simulink model "ZT_VehCtrl_18B"  (R2018b)
settings: Solver=FixedStepAuto  StartTime=0.0  StopTime=inf  FixedStep=0.005  RelTol=1e-3
InitFcn:
  | mbd_mpc_consistency_checks(bdroot(gcs));
undefined symbols (not defined in the file): ANG_DEAD, BMS_NormalPwr, BrkPrsByBrkPct_TB_X, BrkPrsByBrkPct_TB_Y, DELAY_DISCHARGE, DELAY_RCUOFF, DRV_BACKWARD, DRV_BRAKE, DRV_FORWARD, DRV_NEUTRAL, DRV_PARK, DRV_UNPARK, DRV_ZEROTURN, EPB_LOCK, EPB_UNLOCK, ExtraLoadPwr, FanOff, fifo_0_vect, fifo_1_vect, HiFanReq, HV_finished, HV_No_Active, HV_POWER_OFF, HV_POWER_ON, HVDown, HVON, KaTLS_v_DrgUp_X_VehSpd, KeFTM_s_Way1OffDlyTime, KeFTM_TK_Way1CoolLv2OffBatTemp, KeFTM_TK_Way1CoolLv2OffMtrTemp, KeFTM_TK_Way1CoolLv2OnBatTemp, KeFTM_TK_Way1CoolLv2OnMtrTemp, KeFTM_TK_Way1CoolLv3OffBatTemp, KeFTM_TK_Way1CoolLv3OffMtrTemp, KeFTM_TK_Way1CoolLv3OnBatTemp, KeFTM_TK_Way1CoolLv3OnMtrTemp, KeFTM_TK_Way1CoolLv4OffBatTemp, KeFTM_TK_Way1CoolLv4OffMtrTemp, KeFTM_TK_Way1CoolLv4OnBatTemp, KeFTM_TK_Way1CoolLv4OnMtrTemp, Kp1, Kp2, LowFanReq, LQFP, MtrPwrFactor_RCU, MtrPwrHighToMidThd, MtrPwrLowToMidThd, MtrPwrMidToHighThd, MtrPwrMidToLowThd, MtrTrqMax, PCT_DEAD, Precharge, PTO_1000, PTO_540, pts1_fifo_0_vect, pts1_fifo_1_vect, pts2_fifo_0_vect, pts2_fifo_1_vect, pts3_fifo_0_vect, pts3_fifo_1_vect ... (+24)
libraries: mbd_mpc574x_ec_toolbox x124, canmsglib x72, simulink x57
(part 11 of 11)

== stateflow chart ZT_VehCtrl_18B/VehCtrl/EnergyManage1/Chart ==
  state HVon [function] [commented out]
    (default) -> (junction 44) [commented out]
    (junction 44) -> (junction 45) [commented out] : [BMS_BatteryState<=Precharge]
    (junction 44) -> (junction 46) [commented out]
    (junction 45) -> (junction 50) [commented out] : {BMS_Maincircuitcommand=HV_POWER_ON;}
    (junction 46) -> (junction 47) [commented out] : [(BMS_BatteryState==HV_finished)]
    (junction 46) -> (junction 48) [commented out] : {BMS_Maincircuitcommand=HV_No_Active;
        | BMS_Attachment1Circuit=HV_No_Active;
        | BMS_Attachment2Circuit=HV_No_Active;
        | cnt=0;}
    (junction 47) -> (junction 49) [commented out] : {BMS_Attachment1Circuit=HV_POWER_ON;
        | BMS_Attachment2Circuit=HV_POWER_ON;
        | RCU_HVOnOffSts = HVON;
        | cnt = cnt + 1;}
    (junction 49) -> (junction 48) [commented out]
    (junction 50) -> (junction 49) [commented out]
    (junction 48) -> (junction 51) [commented out]
  state PowerOff
    en,du:VCU_Maincircuitcommand = 2; cnt = cnt + 1;
    MCU_Enable = false; MCU_Discharge=true;DCDC_Enable = false;
    VCU_HVOnOffSts = HVDown;
    VCU_RexActiveDischgCmd= true;
    VCU_RexEnableCmd=false;
    VCU_RexStartStopReq=false;
    VCU_FanStsReg=0;
    VCU_MotwaterPumpDutyRe=0;
    Flag=3；
  state init
    en:Ready= false;
    VCU_Maincircuitcommand = 0;
    MCU_Enable = false; MCU_Discharge=false; DCDC_Enable = false;
    VCU_HVOnOffSts = HVON;
    VCU_RexActiveDischgCmd= false;
    VCU_RexEnableCmd=false;
    VCU_RexStartStopReq=false;
    VCU_FanStsReg=0;
    VCU_MotwaterPumpDutyRe=0;
    Flag=0;
  state PowerOn
    state BatChrgSt
      state Discharge
        en,du:
        Flag=5;cnt=cnt+1;
        Ready=false;
        DCDC_Enable = true;
        VCU_RexStartStopReq = false;
        VCU_ReqRexGenPwr = 0;
        VCU_RexEnableCmd= false;
        MCU_Enable = false;
        MCU_Discharge=true;
      state BatChrg
        en,du:
        Flag=6;
        Ready=false;
        DCDC_Enable = true;
        VCU_RexStartStopReq = false;
        VCU_ReqRexGenPwr = 0;
        VCU_RexEnableCmd= false;
        MCU_Enable = false;
        MCU_Discharge=false;
      (default) -> Discharge
      Discharge -> BatChrg : [cnt>DELAY_DISCHARGE]
    state HV_ON
      en:VCU_Maincircuitcommand = 1;
      Flag=1；
    state READY
      en:Ready=true;MCU_Enable = true; DCDC_Enable = true; Flag=2；
      VCU_RexStartStopReq = false;
      VCU_ReqRexGenPwr = 0;
      VCU_RexEnableCmd= false;
    state RCU
      state RCUAuto
        en:Flag=4;VCU_RexStartStopReq = false;
        VCU_ReqRexGenPwr = 0;
        VCU_RexEnableCmd= true;%默认不启动
        du:RcuAuto();
      state RCUOn
        en:Flag=3;
        du:VCU_RexEnableCmd= true;
        VCU_RexStartStopReq=true;
        VCU_ReqRexGenPwr = RCU_RexGenPwr;
        RcuCool();
      (default) -> RCUAuto
      RCUOn -> RCUAuto : [Rcuswitch==0]
      RCUAuto -> RCUOn : [Rcuswitch==1]
    (default) -> HV_ON
    HV_ON -> READY : [BMS_BatteryState==3]
    READY -> BatChrgSt [order 1] : [ChrgSig==1]{cnt = 0;}
    BatChrgSt -> READY : [ChrgSig==0]
    READY -> RCU [order 2] : [(RCU_RexSelfChkSt > 0) && (RCU_RexFltLvl==0)&&(Rcuswitch==0||Rcuswitch==1)]
    RCU -> READY [order 1] : [Rcuswitch==2]
    RCU -> BatChrgSt [order 2] : [ChrgSig==1]{cnt = 0;}
  state HVdown [function] [commented out]
    (default) -> (junction 157) [commented out]
    (junction 157) -> (junction 156) [commented out] : [cnt<DELAY_RCUOFF]
    (junction 157) -> (junction 155) [commented out]
    (junction 156) -> (junction 154) [commented out] : {RCU_RexEnableCmd = false;
        | MCU_Enable = false;
        | DCDC_Enable = false;
        | DCAC_Enable = false;}
    (junction 155) -> (junction 170) [commented out] : [cnt<DELAY_RCUOFF*2]
    (junction 155) -> (junction 168) [commented out] : {MCU_Discharge = true;
        | RCU_RexActiveDischgCmd = true;}
    (junction 170) -> (junction 171) [commented out] : {BMS_Maincircuitcommand=HV_POWER_OFF;
        | BMS_Attachment1Circuit=HV_POWER_OFF;
        | BMS_Attachment2Circuit=HV_POWER_OFF;}
    (junction 171) -> (junction 168) [commented out]
    (junction 154) -> (junction 171) [commented out]
    (junction 168) -> (junction 176) [commented out]
  state RcuAuto [function]
    (default) -> (junction 75) : {VCU_RexEnableCmd= true;} % 高压使能
    (junction 75) -> (junction 76) [order 1] : [(BMS_SOC<35) || (MCU_TotalPwrCmd > BMS_NormalPwr)] % 超功率或亏电，则启动增程器
    (junction 75) -> (junction 78) [order 2]
    (junction 76) -> (junction 74) : {VCU_RexStartStopReq = true;
        |  VCU_ReqRexGenPwr = RCU_RexGenPwr;}
    (junction 78) -> (junction 79) [order 1] : [(BMS_SOC>60) && (MCU_TotalPwrCmd < BMS_NormalPwr)] % 电量充足或低功率，则关闭增程器
    (junction 78) -> (junction 70) [order 2]
    (junction 79) -> (junction 80) : {VCU_RexStartStopReq = false;
        | VCU_ReqRexGenPwr = 0;}
    (junction 80) -> (junction 70)
    (junction 74) -> (junction 80)
    (junction 70) -> (junction 116) : {VCU_MotwaterPumpDutyRe = 100;} % 水泵默认工作
    (junction 116) -> (junction 118) [order 1] : [(RCU_GCUISGInverterTempHiAlarm>0) && (RCU_GCUISGMotorTempHiAlarm>0)] % 双过温，则高速风扇
    (junction 116) -> (junction 128) [order 2]
    (junction 118) -> (junction 126) : {VCU_FanStsReg = HiFanReq;}
    (junction 128) -> (junction 122) [order 1] : [(RCU_GCUISGInverterTempHiAlarm>0) || (RCU_GCUISGMotorTempHiAlarm>0)] % 单过温，则低速风扇
    (junction 128) -> (junction 121) [order 2] : {VCU_FanStsReg = FanOff;} % 未过温，则关闭风扇
    (junction 122) -> (junction 125) : {VCU_FanStsReg = LowFanReq;}
    (junction 125) -> (junction 121)
    (junction 126) -> (junction 125)
    (junction 121) -> (junction 130)
  state RcuCool [function]
    (default) -> (junction 269) : {VCU_MotwaterPumpDutyRe = 100;} % 水泵默认工作
    (junction 269) -> (junction 270) [order 1] : [(RCU_GCUISGInverterTempHiAlarm>0) && (RCU_GCUISGMotorTempHiAlarm>0)] % 双过温，则高速风扇
    (junction 269) -> (junction 271) [order 2]
    (junction 270) -> (junction 275) : {VCU_FanStsReg = HiFanReq;}
    (junction 271) -> (junction 272) [order 1] : [(RCU_GCUISGInverterTempHiAlarm>0) || (RCU_GCUISGMotorTempHiAlarm>0)] % 单过温，则低速风扇
    (junction 271) -> (junction 273) [order 2] : {VCU_FanStsReg = FanOff;} % 未过温，则关闭风扇
    (junction 272) -> (junction 274) : {VCU_FanStsReg = LowFanReq;}
    (junction 274) -> (junction 273)
    (junction 275) -> (junction 274)
    (junction 273) -> (junction 276)
  (default) -> init
  PowerOff -> init : [(cnt>DELAY_DISCHARGE)&&(BMS_BatteryState==4)]
  init -> PowerOn : [(Key>0) && ShutDown==0]
  PowerOn -> PowerOff : [(Key==0) || ShutDown>0]{cnt = 0;}
  data: Key input; ShutDown input; HV_No_Active parameter double; HV_POWER_ON parameter; HV_POWER_OFF parameter; cnt local single =single(0); VCU_Maincircuitcommand output uint8; VCU_HVOnOffSts output uint8; VCU_RexEnableCmd output boolean; VCU_RexStartStopReq output boolean; VCU_ReqRexGenPwr output single =single(-60); VCU_FanStsReg output uint8; VCU_MotwaterPumpDutyRe output single; VCU_RexActiveDischgCmd output boolean; HVON parameter; HVDown parameter; FanOff parameter; LowFanReq parameter; RCU_RexSelfChkSt input; RCU_RexFltLvl input; RCU_RexGenPwrMaxLim input; RCU_GCUISGInverterTempHiAlarm input; RCU_GCUISGMotorTempHiAlarm input; MCU_TotalPwrCmd input; HiFanReq parameter; DELAY_RCUOFF parameter; DELAY_DISCHARGE parameter; MCU_Enable output boolean; MCU_Discharge output boolean; BMS_SOC input; BMS_NormalPwr parameter; BMS_BatteryState input; ChrgSig input; Ready output; DCDC_Enable output; Precharge parameter; HV_finished parameter; Flag output; Rcuswitch input; MtrPwrHighToMidThd parameter; MtrPwrLowToMidThd parameter; MtrPwrMidToHighThd parameter; MtrPwrMidToLowThd parameter; RexGenPwrHigh parameter; RexGenPwrLow parameter; RexGenPwrMid parameter; RCU_RexGenPwr input

== stateflow chart ZT_VehCtrl_18B/VehCtrl/FaultProc/Subsystem5/TimeOutLevel_RMT1 ==
  state on
    en:TimeOutLevel=1;LifeTemp=LiveCounter;
    du:LifeTemp=LiveCounter;
  state on_cnt
    en:TimeOutLevel=1;cnt=0;
    du:cnt = cnt + 1;
  state off
    en:TimeOutLevel=0;
  (default) -> on
  on -> on_cnt : [LiveCounter==LifeTemp]
  on_cnt -> on [order 2] : [LiveCounter~=LifeTemp]
  off -> on : [LiveCounter~=LifeTemp]
  on_cnt -> off [order 1] : [(cnt>=10)]
  data: LiveCounter input; TimeOutLevel output; LifeTemp local; cnt local

== stateflow chart ZT_VehCtrl_18B/VehCtrl/FaultProc/Subsystem5/PacketLoss_RMT ==
  state on
    en:PacketLossFlg=0;
  state on_cnt
    en:PacketLossFlg=0;cnt=0;
    du:cnt = cnt + 1;
  state off
    en:PacketLossFlg=1;
  (default) -> on
  on -> on_cnt : [(PacketLoss==1)||(CheckSum==1)]
  on_cnt -> on [order 2] : [(PacketLoss==0)&(CheckSum==0)]
  off -> on : [(PacketLoss==0)&(CheckSum==0)]
  on_cnt -> off [order 1] : [(cnt>=10)]
  data: CheckSum input; PacketLossFlg output; cnt local; PacketLoss input

== stateflow chart ZT_VehCtrl_18B/VehCtrl/FaultProc/Subsystem5/PacketLoss_RMT1 ==
  state on
    en:PacketLossFlg=0;
  state on_cnt
    en:PacketLossFlg=0;cnt=0;
    du:cnt = cnt + 1;
  state off
    en:PacketLossFlg=1;
  (default) -> on
  on -> on_cnt : [(PacketLoss==1)||(CheckSum==1)]
  on_cnt -> on [order 2] : [(PacketLoss==0)&(CheckSum==0)]
  off -> on : [(PacketLoss==0)&(CheckSum==0)]
  on_cnt -> off [order 1] : [(cnt>=10)]
  data: CheckSum input; PacketLossFlg output; cnt local; PacketLoss input

== stateflow chart ZT_VehCtrl_18B/VehCtrl/FaultProc/Subsystem5/TimeOutLevel_RMT ==
  state on
    en:TimeOutLevel=1;LifeTemp=LiveCounter;
    du:LifeTemp=LiveCounter;
  state on_cnt
    en:TimeOutLevel=1;cnt=0;
    du:cnt = cnt + 1;
  state off
    en:TimeOutLevel=0;
  (default) -> on
  on -> on_cnt : [LiveCounter==LifeTemp]
  on_cnt -> on [order 2] : [LiveCounter~=LifeTemp]
  off -> on : [LiveCounter~=LifeTemp]
  on_cnt -> off [order 1] : [(cnt>=10)]
  data: LiveCounter input; TimeOutLevel output; LifeTemp local; cnt local

== stateflow chart ZT_VehCtrl_18B/SigOut/GPIO /PWM_OUT/FreqCMD ==
  settings: executeAtInitialization=1
  state A
    du:
    freq = 20000;
    cntr = cntr + 1;
    dc = 0.25;
  state A1
    du:
    freq = 10000;
    cntr = cntr - 1;
    dc =  0.5;
  (default) -> A : {cntr=0;dc=0;}
  A1 -> A : [cntr < 1]
  A -> A1 : [cntr > 50]
  data: cntr local uint32 =0; freq output uint32; dc output single

== stateflow chart ZT_VehCtrl_18B/VehCtrl/TempertureControl/ThermFR_RRvRead1/Way1_Cool_Level ==
  settings: executeAtInitialization=1
  state Ready
    state Level_1
      en:
      MtrPumpLv=1;
      Fan_Low=0;
    state Level_2
      en:
      MtrPumpLv=2;
      Fan_Low=1;
    state Level_4
      en:
      MtrPumpLv=4;
      Fan_Low=0;
    state Level_3
      en:
      MtrPumpLv=3;
      Fan_Low=1;
    Level_1 -> Level_2 : [Temp>=Ke_Lv2OnTemp]
    (default) -> Level_1
    Level_2 -> Level_1 [order 1] : [Temp<=Ke_Lv2OffTemp]
    Level_2 -> Level_3 [order 2] : [Temp>=Ke_Lv3OnTemp]
    Level_3 -> Level_2 [order 1] : [Temp<=Ke_Lv3OffTemp]
    Level_3 -> Level_4 [order 2] : [Temp>=Ke_Lv4OnTemp]
    Level_4 -> Level_3 : [Temp<=Ke_Lv4OffTemp]
  state Level_0
    en:
    MtrPumpLv=0;
    Fan_Low=0;
  state OFF_Cnt
    en:
    Cnt=1;
    du:
    Cnt++;
  (default) -> Level_0
  Level_0 -> Ready : [RdySt==1]
  OFF_Cnt -> Level_0 : [Cnt>=Ke_OffDlyCnt]
  Ready -> OFF_Cnt : [RdySt==0]
  data: RdySt input; Temp input; Ke_Lv2OffTemp input; Ke_Lv2OnTemp input; Ke_Lv3OffTemp input; Ke_Lv3OnTemp input; Ke_Lv4OffTemp input; Ke_Lv4OnTemp input; Ke_OffDlyCnt input; Cnt local uint32; Fan_Low output uint8; MtrPumpLv output double

== stateflow chart ZT_VehCtrl_18B/Initialization & SPI timer1/CS1 LS/Chart ==
  state clear
    en:high=128+7;low=1;cnt=0;
    du:cnt = cnt + 1;
  state en
    en:high=128+1+64;low=0;cnt=0;
    du:cnt = cnt + 1;
  state config
    en:high=128+7+64;low=1+128;cnt=0;
    du:cnt = cnt + 1;
  (default) -> clear
  clear -> en : [cnt>5]
  en -> config : [cnt>5]
  data: high output; low output; cnt local

== stateflow chart ZT_VehCtrl_18B/VehCtrl/TempertureControl/ThermLvRead3/Way1_Cool_Level ==
  settings: executeAtInitialization=1
  state Ready
    state Level_2
      en:
      MtrPumpLv=2;
      Fan_Low=1;
      Fan_High=0;
      V1 = 1; V2 = 1; V3 = 0; V4 = 0;
    state Level_1
      en:
      MtrPumpLv=1;
      Fan_Low=0;
      Fan_High=0;
      V1 = 1; V2 = 0; V3 = 0; V4 = 0;
    state Level_4
      en:
      MtrPumpLv=4;
      Fan_Low=0;
      Fan_High=1;
      V1 = 1; V2 = 1; V3 = 1; V4 = 1;
    state Level_3
      en:
      MtrPumpLv=3;
      Fan_Low=0;
      Fan_High=1;
      V1 = 1; V2 = 1; V3 = 1; V4 = 0;
    Level_1 -> Level_2 : [Temp>=Ke_Lv2OnTemp]
    (default) -> Level_1
    Level_2 -> Level_1 [order 1] : [Temp<=Ke_Lv2OffTemp]
    Level_2 -> Level_3 [order 2] : [Temp>=Ke_Lv3OnTemp]
    Level_3 -> Level_2 [order 1] : [Temp<=Ke_Lv3OffTemp]
    Level_3 -> Level_4 [order 2] : [Temp>=Ke_Lv4OnTemp]
    Level_4 -> Level_3 : [Temp<=Ke_Lv4OffTemp]
  state Level_0
    en:
    MtrPumpLv=0;
    Fan_Low=0;
    Fan_High=0;
    V1 = 0; V2 = 0; V3 = 0; V4 = 0;
  state OFF_Cnt
    en:
    Cnt=1;
    du:
    Cnt++;
  (default) -> Level_0
  Level_0 -> Ready : [RdySt==1]
  OFF_Cnt -> Level_0 : [Cnt>=Ke_OffDlyCnt]
  Ready -> OFF_Cnt : [RdySt==0]
  data: RdySt input; Temp input; Ke_Lv2OffTemp input; Ke_Lv2OnTemp input; Ke_Lv3OffTemp input; Ke_Lv3OnTemp input; Ke_Lv4OffTemp input; Ke_Lv4OnTemp input; Ke_OffDlyCnt input; Cnt local uint32; Fan_Low output uint8; Fan_High output uint8; V1 output double; V2 output double; V3 output double; V4 output double; MtrPumpLv output uint8

== stateflow chart ZT_VehCtrl_18B/VehCtrl/LedControl/Chart ==
  state Normal
    state Turn_Right
      state LightOn
        Right_Cmd=1;
      state LightOff
        Right_Cmd=0;
      (default) -> Normal.Turn_Right.LightOn
      Normal.Turn_Right.LightOff -> Normal.Turn_Right.LightOn : [after(0.5,sec)]
      Normal.Turn_Right.LightOn -> Normal.Turn_Right.LightOff : [after(0.5,sec)]
    state Neutral
      en:
      Left_Cmd=0;
      Right_Cmd=0;
    state Turn_Left
      state LightOn
        Left_Cmd=1;
      state LightOff
        Left_Cmd=0;
      (default) -> Normal.Turn_Left.LightOn
      Normal.Turn_Left.LightOff -> Normal.Turn_Left.LightOn : [after(0.5,sec)]
      Normal.Turn_Left.LightOn -> Normal.Turn_Left.LightOff : [after(0.5,sec)]
    Neutral -> Turn_Right [order 1] : [SteerAng>=DeadBand1]
    (default) -> Neutral
    Turn_Right -> Neutral : [SteerAng<DeadBand2]
    Turn_Left -> Neutral : [SteerAng>-DeadBand2]
    Neutral -> Turn_Left [order 2] : [SteerAng<=-DeadBand1]
  state SOCmode
    state LightOn
      Right_Cmd=1;
      Left_Cmd=1;
    state LightOff
      Right_Cmd=0;
      Left_Cmd=0;
    (default) -> SOCmode.LightOn
    SOCmode.LightOff -> SOCmode.LightOn : [after(0.5,sec)]
    SOCmode.LightOn -> SOCmode.LightOff : [after(0.5,sec)]
  (default) -> Normal
  SOCmode -> Normal : [soc>35]
  Normal -> SOCmode : [soc<30]
  data: soc input; SteerAng input; DeadBand1 local =3; DeadBand2 local =2; Left_Cmd output; Right_Cmd output

== stateflow chart ZT_VehCtrl_18B/Initialization & SPI timer1/CS3 LS/Chart ==
  state ConfigA
    en:high=80+mode*(1+4);low=0+mode*(1+4);cnt=0;
    du:cnt = cnt + 1;
  state en
    en:high=96;low=0;cnt=0;
  (default) -> ConfigA
  ConfigA -> en : [cnt>4]
  data: high output; low output; cnt local; mode input

== stateflow chart ZT_VehCtrl_18B/VehCtrl/TempertureControl/ThermFR_RRvRead2/Way1_Cool_Level ==
  settings: executeAtInitialization=1
  state Ready
    state Level_1
      en:
      MtrPumpLv=1;
      Fan_Low=0;
    state Level_2
      en:
      MtrPumpLv=2;
      Fan_Low=1;
    state Level_4
      en:
      MtrPumpLv=4;
      Fan_Low=0;
    state Level_3
      en:
      MtrPumpLv=3;
      Fan_Low=1;
    Level_1 -> Level_2 : [Temp>=Ke_Lv2OnTemp]
    (default) -> Level_1
    Level_2 -> Level_1 [order 1] : [Temp<=Ke_Lv2OffTemp]
    Level_2 -> Level_3 [order 2] : [Temp>=Ke_Lv3OnTemp]
    Level_3 -> Level_2 [order 1] : [Temp<=Ke_Lv3OffTemp]
    Level_3 -> Level_4 [order 2] : [Temp>=Ke_Lv4OnTemp]
    Level_4 -> Level_3 : [Temp<=Ke_Lv4OffTemp]
  state Level_0
    en:
    MtrPumpLv=0;
    Fan_Low=0;
  state OFF_Cnt
    en:
    Cnt=1;
    du:
    Cnt++;
  (default) -> Level_0
  Level_0 -> Ready : [RdySt==1]
  OFF_Cnt -> Level_0 : [Cnt>=Ke_OffDlyCnt]
  Ready -> OFF_Cnt : [RdySt==0]
  data: RdySt input; Temp input; Ke_Lv2OffTemp input; Ke_Lv2OnTemp input; Ke_Lv3OffTemp input; Ke_Lv3OnTemp input; Ke_Lv4OffTemp input; Ke_Lv4OnTemp input; Ke_OffDlyCnt input; Cnt local uint32; Fan_Low output uint8; MtrPumpLv output double

== stateflow chart ZT_VehCtrl_18B/VehCtrl/LedControl/Chart1 ==
  state unNormal
    en,du:Green=0;Red=1；
  state Normal
    state RMT
      en,du:Green=1;Red=0;
    state Auto
      en,du:Green=1;Red=1;%黄色
    (default) -> RMT
    RMT -> Auto : [CtrMode==1]
    Auto -> RMT : [CtrMode==0]
  (default) -> Normal
  Normal -> unNormal : [Fault>0]
  unNormal -> Normal : [Fault==0]
  data: CtrMode input; Fault input; Red output; Green output

== stateflow chart ZT_VehCtrl_18B/VehCtrl/MontionControl/ValveControl/SteerSys/Chart ==
  state Left
    en,du:flg=1;
  state Hold
    en,du:flg=0;
  state Right
    en,du:flg=2;
  (default) -> Hold
  Hold -> Left [order 1] : [StrErr>0.7]
  Left -> Hold : [StrErr<=0.5]
  Hold -> Right [order 2] : [StrErr<-0.7]
  Right -> Hold : [StrErr>-0.4]
  data: StrErr input; flg output

== stateflow chart ZT_VehCtrl_18B/VehCtrl/MontionControl/DriveControl/DriveModeTrans ==
  state Park [commented out]
    en,du:VehDrv=0;SpdTgt=0;VehBrk=CmdBrk;
    state Lock [commented out]
      en,du:EpbSt = EPB_LOCK;DrvPhase = DRV_PARK;cnt=0;
    state Unlock [commented out]
      en:EpbSt = EPB_UNLOCK;DrvPhase = DRV_UNPARK;cnt=0;
      du:VehBrk=CmdBrk;cnt = cnt + 1;
    (default) -> Lock [commented out]
    Lock -> Unlock [commented out] : [(CmdPark==EPB_UNLOCK)...
        |  || ((CmdDrv>PCT_DEAD)&&(CmdBrk<=0.5*PCT_DEAD))...
        |  || (CmdSpd>SPD_DEAD)]
        | % 释放驻车请求，或踩油门，或车速请求
    Unlock -> Lock [commented out] : [(CmdPark==EPB_LOCK)]
        | % 驻车请求
  state Run
    state TrqCtrl
      en:VehBrk=0;ModeSpd=false;SpdTgt=0;
      state Normal
        state Backward
          en,du:VehDrv=CmdDrv;DrvPhase = DRV_BACKWARD;
        state Forward
          en,du:VehDrv=CmdDrv;DrvPhase = DRV_FORWARD;
        state Neutral
          en:VehDrv=0;DrvPhase = DRV_NEUTRAL; % 预留再生制动
        Run.TrqCtrl.Normal.Neutral -> Forward [order 2] : [(VehSpd>=-1*SPD_DEAD) && ModeDirection==0]
            | % 前进挡及非倒车状态
        Forward -> Run.TrqCtrl.Normal.Neutral : [ModeDirection>0]
            | % 换挡
        Run.TrqCtrl.Normal.Neutral -> Backward [order 1] : [(VehSpd<=SPD_DEAD) && ModeDirection>0]
            | % 后退挡及非前进状态
        Backward -> Run.TrqCtrl.Normal.Neutral : [ModeDirection==0]
            | % 换挡
        (default) -> Run.TrqCtrl.Normal.Neutral
      state ZeroTurn
        en:VehDrv=CmdDrv;DrvPhase = DRV_ZEROTURN;
      (default) -> Normal
      Normal -> Run.TrqCtrl.ZeroTurn : [(ModeSteer>0)&&(StrReady>0)]
          | % 原地转向请求且已完成准备
      Run.TrqCtrl.ZeroTurn -> Normal : [ModeSteer==0]
          | % 常规转向请求
    state SpdCtrl [commented out]
      en:VehBrk=0;ModeSpd=true;VehDrv=0;
      state Neutral [commented out]
        en:SpdTgt=CmdSpd;DrvPhase = DRV_NEUTRAL; % 预留再生制动
      state ZeroTurn [commented out]
        en:SpdTgt=0;DrvPhase = DRV_ZEROTURN;
      (default) -> Run.SpdCtrl.Neutral [commented out]
      Run.SpdCtrl.Neutral -> Run.SpdCtrl.ZeroTurn [commented out] : [(ModeSteer>0) && (StrReady>0)]
          | % 原地转向请求且已完成准备
      Run.SpdCtrl.ZeroTurn -> Run.SpdCtrl.Neutral [commented out] : [ModeSteer==0]
          | % 常规转向请求
    (default) -> TrqCtrl
    TrqCtrl -> SpdCtrl [commented out] : [(ModeDrive>0)]
        | % [(abs(VehSpd)<=SPD_DEAD)&&(ModeDrive>0)]
        | % 车速控制请求及车辆静止
    SpdCtrl -> TrqCtrl [commented out] : [(ModeDrive==0)]
        | % [(abs(VehSpd)<=SPD_DEAD)&&(ModeDrive==0)]
        | % 转矩控制请求及车辆静止
  state Brake
    en,du:VehDrv=0;SpdTgt=0;VehBrk=CmdBrk;DrvPhase = DRV_BRAKE;
  (default) -> Run
  Park -> Run [commented out] : [(cnt>=10)]
      | % 已释放驻车
  Run -> Park [commented out] : [(VehSpd<=SPD_DEAD)&&(CmdPark==EPB_LOCK)]
      | % 驻车请求及车辆静止
  Brake -> Park [commented out] : [(VehSpd<=SPD_DEAD)&&(CmdPark==EPB_LOCK)]
      | % 驻车请求及车辆静止
  Run -> Brake : [CmdBrk>PCT_DEAD]
      | % 有制动
  Brake -> Run : [CmdBrk<=0.5*PCT_DEAD && (ModeDrive==0)]
      | % 松制动
  data: CmdDrv input; CmdBrk input; ModeDrive input; CmdPark input; ModeDirection input; ModeSteer input; CmdSpd input; StrReady input; VehBrk output single =single(0); EpbSt output uint8 =uint8(0); VehDrv output single =single(0); VehSpd input; EPB_LOCK parameter; EPB_UNLOCK parameter; PCT_DEAD parameter; SPD_DEAD parameter; SpdTgt output single =single(0); ModeSpd output boolean =false; DrvPhase output uint8 =uint8(0); cnt local single =single(0); DRV_PARK parameter; DRV_UNPARK parameter; DRV_BRAKE parameter; DRV_NEUTRAL parameter; DRV_FORWARD parameter; DRV_BACKWARD parameter; DRV_ZEROTURN parameter

== stateflow chart ZT_VehCtrl_18B/VehCtrl/MontionControl/ValveControl/SteerSys/Chart1 ==
  state Hold
    en,du:u=0;flg=0;
  state Ctrl
    en,du:flg=1;u=AngCmdFF;
  (default) -> Hold
  Hold -> Ctrl : [abs(AngCmd-AngRel)>STR_CTRLDEAD]
  Ctrl -> Hold : [abs(AngCmd-AngRel)<=0.5*STR_CTRLDEAD]
  data: AngCmdFF input; AngCmd input; AngRel input; u output; flg output; STR_CTRLDEAD parameter

== stateflow chart ZT_VehCtrl_18B/Initialization & SPI timer1/CS5 LS/Chart ==
  state clear
    en:high=128+7;low=1;cnt=0;
    du:cnt = cnt + 1;
  state en
    en:high=128+1+64;low=0;cnt=0;
    du:cnt = cnt + 1;
  state config
    en:high=128+7+64;low=1+128;cnt=0;
  (default) -> clear
  clear -> en : [cnt>5]
  en -> config : [cnt>5]
  data: high output; low output; cnt local

== stateflow chart ZT_VehCtrl_18B/Initialization & SPI timer1/Chart ==
  state Idle
    en:Flg=0;
  state Initialize
    en:Flg=1;
  state Normal
    en:Flg=2;
  (default) -> Idle
  Normal -> Idle : [ResetFlg==1]
  Initialize -> Idle [order 2] : [ResetFlg==1]
  Idle -> Initialize : [ResetFlg==0]
  Initialize -> Normal [order 1] : [InitFlg>0]
  data: ResetFlg input; InitFlg input; Flg output

== stateflow chart ZT_VehCtrl_18B/Initialization & SPI timer1/Chart1 ==
  state IDLE
    en:Flg=0;
  state CS1
    en:Flg=1;cnt=0;
    du:cnt = cnt + 1;
  state CS5
    en:Flg=2;cnt=0;
    du:cnt = cnt + 1;
  state Done
    en:Flg=9;
  (default) -> IDLE
  Done -> IDLE : [VcuMode==0]
  IDLE -> CS1 : [VcuMode==1]
  CS1 -> CS5 : [cnt>20]
  CS5 -> Done : [cnt>20]
  data: VcuMode input; Flg output; cnt local

== stateflow chart ZT_VehCtrl_18B/Initialization & SPI timer1/Chart2 ==
  state IDLE
    en:Flg=0;
  state CS2
    en:Flg=1;cnt=0;
    du:cnt = cnt + 1;
  state CS3
    en:Flg=2;cnt=0;
    du:cnt = cnt + 1;
  state Done
    en:Flg=9;
  (default) -> IDLE
  Done -> IDLE : [VcuMode==0]
  IDLE -> CS2 : [VcuMode==1]
  CS2 -> CS3 : [cnt>20]
  CS3 -> Done : [cnt>20]
  data: VcuMode input; Flg output; cnt local

== stateflow chart ZT_VehCtrl_18B/VehCtrl/MontionControl/DriveControl/Motor/WheelControl/Chart ==
  (default) -> (junction 14)
  (junction 14) -> (junction 15) [order 1] : [DrvPhase==DRV_ZEROTURN] % 原地转向
  (junction 14) -> (junction 16) [order 2] : {
      | MtrTrq = VehTrq/Ratio/4;
      | MtrTrqCmdFL = MtrTrq;
      | MtrTrqCmdFR = MtrTrq;
      | MtrTrqCmdRL = MtrTrq;
      | MtrTrqCmdRR = MtrTrq;
      | }
  (junction 15) -> (junction 35) : {
      | MtrTrq = abs(CmdStrAng)/StrAngMax * MtrTrqZeroturn;
      | }
  (junction 16) -> (junction 17) [order 1] : [DrvPhase==DRV_BACKWARD] % 倒车
  (junction 35) -> (junction 39) [order 1] : [CmdStrAng>0] % 左转
  (junction 16) -> (junction 18) [order 2] : % 默认前进
      | {
      | MtrDirCmdFL = false;
      | MtrDirCmdFR = false;
      | MtrDirCmdRL = false;
      | MtrDirCmdRR = false;
      | }
  (junction 17) -> (junction 19) : {
      | MtrDirCmdFL = true;
      | MtrDirCmdFR = true;
      | MtrDirCmdRL = true;
      | MtrDirCmdRR = true;
      | }
  (junction 35) -> (junction 34) [order 2] : {
      | MtrTrqCmdFL = MtrTrq*FacFrontOuter;
      | MtrTrqCmdFR = MtrTrq*FacFrontInter;
      | MtrTrqCmdRL = MtrTrq*FacRearOuter;
      | MtrTrqCmdRR = MtrTrq*FacRearInter;
      | MtrDirCmdFL = false;
      | MtrDirCmdFR = true;
      | MtrDirCmdRL = false;
      | MtrDirCmdRR = true;
      | }
  (junction 39) -> (junction 33) : {
      | MtrTrqCmdFL = MtrTrq*FacFrontInter;
      | MtrTrqCmdFR = MtrTrq*FacFrontOuter;
      | MtrTrqCmdRL = MtrTrq*FacRearInter;
      | MtrTrqCmdRR = MtrTrq*FacRearOuter;
      | MtrDirCmdFL = true;
      | MtrDirCmdFR = false;
      | MtrDirCmdRL = true;
      | MtrDirCmdRR = false;
      | }
  (junction 19) -> (junction 18)
  (junction 34) -> (junction 19)
  (junction 33) -> (junction 34)
  (junction 18) -> (junction 21) : {
      | MtrTrqCmdFL = min(MtrTrqCmdFL, TrqMax);
      | MtrTrqCmdFR = min(MtrTrqCmdFR, TrqMax);
      | MtrTrqCmdRL = min(MtrTrqCmdRL, TrqMax);
      | MtrTrqCmdRR = min(MtrTrqCmdRR, TrqMax);
      | }
  data: MtrDirCmdFL output boolean; MtrDirCmdFR output boolean; MtrDirCmdRL output boolean; MtrDirCmdRR output boolean; DrvPhase input; VehTrq input; TrqMax input; CmdStrAng input; MtrTrqCmdFL output; MtrTrqCmdFR output; MtrTrqCmdRL output; MtrTrqCmdRR output; MtrTrq local; Ratio parameter; StrAngMax parameter; MtrTrqZeroturn input; DRV_ZEROTURN parameter; DRV_BACKWARD parameter; FacFrontInter input; FacFrontOuter input; FacRearInter input; FacRearOuter input

== stateflow chart ZT_VehCtrl_18B/VehCtrl/MontionControl/SteerControl/Chart ==
  state Ackermann
    state Corner
      en,du:StrPhase=STR_ACKERMANN;
      AngCmdOut=AngCmd;
    state Straight
      en,du:StrPhase=STR_STRAIGHT;AngCmdOut=0;
    (default) -> Straight
    Straight -> Corner : [abs(AngCmd)>=ANG_DEAD]
    Corner -> Straight : [abs(AngCmd)<0.5*ANG_DEAD]
  state Zero_turn
    en,du:StrPhase=STR_ZERO;
  (default) -> Ackermann
  Ackermann -> Zero_turn : [(abs(VehSpd)<=SPD_DEAD)&&(Mode>0)]
  Zero_turn -> Ackermann : [(abs(VehSpd)<=SPD_DEAD)&&Mode==0]
  data: VehSpd input; Mode input; AngCmd input; Ang input; AngCmdOut output single; StrPhase output uint8; STR_STRAIGHT parameter; STR_ACKERMANN parameter; STR_ZERO parameter; STR_ACK2ZERO parameter; STR_ZERO2ACK parameter; ANG_DEAD parameter; SPD_DEAD parameter

== stateflow chart ZT_VehCtrl_18B/VehCtrl/MontionControl/ValveControl/BrakeSys/Chart ==
  state Decrease
    during:
    BrkValve = brakecontrol(BrkPrsTgt,BrkPrs);
  state ldle
    during:
    BrkValve = BrkValve;  % 保持不变
  state Increase
    during:
    BrkValve = brakecontrol(BrkPrsTgt,BrkPrs);
  (default) -> ldle
  ldle -> Decrease [order 1] : [BrkPrsTgt < BrkPrs - deadband]
  ldle -> Increase [order 2] : [BrkPrsTgt > BrkPrs + deadband]
  Increase -> ldle : [abs(BrkPrsTgt - BrkPrs) <= deadband]
  Decrease -> ldle : [abs(BrkPrsTgt - BrkPrs) <= deadband]
  data: brk_prstgt function_input; brk_prs function_input; breakvalue function_output; Ts function_input; deadband local double =10; BrkPrs input; BrkPrsTgt input; BrkValve output double
  function breakvalue = brakecontrol(brk_prstgt, brk_prs, Ts):
    | function breakvalue = brakecontrol(brk_prstgt, brk_prs, Ts)
    | % BRAKE_CONTROL_PID 刹车压力闭环PID控制函数 (Matlab 实现)
    | %
    | % 输入:
    | %   brk_prstgt: 期望刹车压力 (0-100%)
    | %   brk_prs:    当前实际刹车压力 (0-100%)
    | %   Ts:         控制周期时间 (秒), 例如 0.01s (10ms)
    | %
    | % 输出:
    | %   valve_output: 刹车阀输出指令 (0-2048, 整数)
    | 
    | % --- 1. 定义 PID 参数 ---
    | % 这些参数需要通过实际系统测试进行整定（Tuning）
    | Kp = 5.0;     % 比例增益 (通常是主导项)
    | Ki = 0.5;     % 积分增益 (消除稳态误差)
    | Kd = 0.01;    % 微分增益 (抑制超调)
    | Ts=0.005;
    | % --- 2. 硬件与比例定义 ---
    | VALVE_MAX = 2048.0;     % 阀门输出最大值
    | SCALE_FACTOR = VALVE_MAX / 100.0; % 比例因子 (2048 / 100 = 20.48)
    | 
    | % --- 3. 持久化状态 (用于积分项和微分项) ---
    | % 使用 persistent 关键字使变量在函数调用结束后仍保持其值
    | persistent integral_term prev_error
    | 
    | % 初始化持久化变量
    | if isempty(integral_term)
    |     integral_term = 0.0;
    |     prev_error = 0.0;
    | end
    | 
    | % --- 4. 核心 PID 计算 ---
    | 
    | % a. 计算误差
    | error = brk_prstgt - brk_prs;
    | 
    | % b. 比例项 (P Term)
    | P_out = Kp * error;
    | 
    | % c. 积分项 (I Term)
    | integral_term = integral_term + error * Ts;
    | 
    | % **防积分饱和 (Anti-windup)**: 限制积分项累积
    | % 限制范围：I_out 的绝对值不能超过 VALVE_MAX
    | integral_max = VALVE_MAX / Ki;
    | if integral_term > integral_max
    |     integral_term = integral_max;
    | elseif integral_term < 0
    |     % 刹车控制通常是单向的（只有压力增加），但为了通用性保留负限幅
    |     integral_term = max(integral_term, -integral_max); 
    | end
    | I_out = Ki * integral_term;
    | 
    | % d. 微分项 (D Term)
    | % 计算误差变化率 (微分)
    | derivative = (error - prev_error) / Ts;
    | D_out = Kd * derivative;
    | 
    | % --- 5. 总输出与限幅 ---
    | 
    | % e. 计算总控制信号 (百分比量纲)
    | control_signal_perc = P_out + I_out + D_out;
    | 
    | % f. 转换为硬件输出量程 (0-2048)
    | breakvalve_raw = control_signal_perc * SCALE_FACTOR;
    | 
    | % g. 硬件输出限幅 (Clamping)
    | if breakvalve_raw > VALVE_MAX
    |     breakvalve_raw = VALVE_MAX;
    | elseif breakvalve_raw < 0.0
    |     breakvalve_raw = 0.0;
    | end
    | 
    | % h. 更新状态
    | prev_error = error;
    | 
    | % --- 6. 返回结果 ---
    | breakvalue = round(breakvalve_raw); % 返回整数指令
    | end

== stateflow chart ZT_VehCtrl_18B/VehCtrl/FaultProc/Subsystem5/TimeOutLevel_RMT2 ==
  state on
    en:TimeOutLevel=1;LifeTemp=LiveCounter;
    du:LifeTemp=LiveCounter;
  state on_cnt
    en:TimeOutLevel=1;cnt=0;
    du:cnt = cnt + 1;
  state off
    en:TimeOutLevel=0;
  (default) -> on
  on -> on_cnt : [LiveCounter==LifeTemp]
  on_cnt -> on [order 2] : [LiveCounter~=LifeTemp]
  off -> on : [LiveCounter~=LifeTemp]
  on_cnt -> off [order 1] : [(cnt>=10)]
  data: LiveCounter input; TimeOutLevel output; LifeTemp local; cnt local

== stateflow chart ZT_VehCtrl_18B/VehCtrl/FaultProc/Subsystem5/PacketLoss_RMT2 ==
  state on
    en:PacketLossFlg=0;
  state on_cnt
    en:PacketLossFlg=0;cnt=0;
    du:cnt = cnt + 1;
  state off
    en:PacketLossFlg=1;
  (default) -> on
  on -> on_cnt : [(PacketLoss==1)||(CheckSum==1)]
  on_cnt -> on [order 2] : [(PacketLoss==0)&(CheckSum==0)]
  off -> on : [(PacketLoss==0)&(CheckSum==0)]
  on_cnt -> off [order 1] : [(cnt>=10)]
  data: CheckSum input; PacketLossFlg output; cnt local; PacketLoss input

== stateflow chart ZT_VehCtrl_18B/VehCtrl/EnergyManage1/Chart1 ==
  state Low
    during:
    RCU_RexGenPwr = RexGenPwrLow;
  state Mid
    during:
    RCU_RexGenPwr = RexGenPwrMid;
  state High
    during:
    RCU_RexGenPwr = RexGenPwrHigh;
  (default) -> Low
  Low -> Mid : [MtrPwrTotal >= MtrPwrLowToMidThd]
  Mid -> Low [order 1] : [MtrPwrTotal <= MtrPwrMidToLowThd]
  Mid -> High [order 2] : [MtrPwrTotal >= MtrPwrMidToHighThd]
  High -> Mid : [MtrPwrTotal <= MtrPwrHighToMidThd]
  data: MtrPwrHighToMidThd parameter; MtrPwrLowToMidThd parameter; MtrPwrMidToHighThd parameter; MtrPwrMidToLowThd parameter; MtrPwrTotal input; RCU_RexGenPwr output; RexGenPwrHigh parameter; RexGenPwrLow parameter; RexGenPwrMid parameter
